simulink model "old_sea_controllers"  (R2012b)
settings: Solver=ode45  StartTime=0.0  StopTime=10.0  RelTol=1e-3
values from neighbouring files (symbols this model uses):
  sample_time = 1/update_freq    (= 0.001)    [init_umich_2d_walking.m]
undefined symbols (not defined in the file or in its folder): DiscIntNeverNeededParam, i_limit_sea_position, k_leg_spring, kd_sea_position, ki_sea_position, ki_sea_torque, kp_sea_position, kp_sea_torque, LEG_MTR_MAX_TORQUE, virtual_spring_damping
settings Model: Creator=wmartin  LastModifiedBy=wmartin

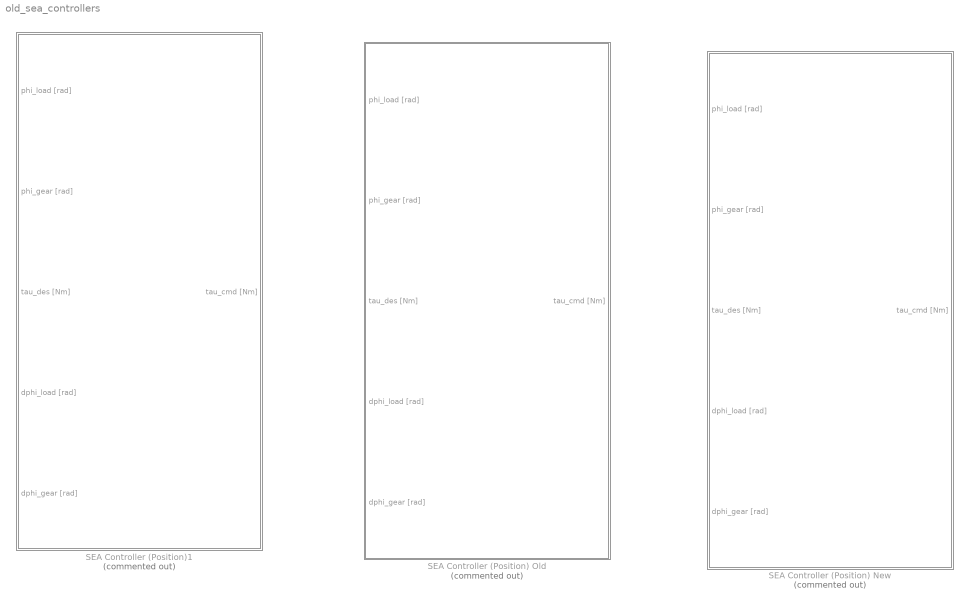
== system old_sea_controllers ==
  SEA Controller (Position) New : Subsystem  Commented=on
  SEA Controller (Position) Old : Subsystem  Commented=on
  SEA Controller (Position)1 : Subsystem  Commented=on

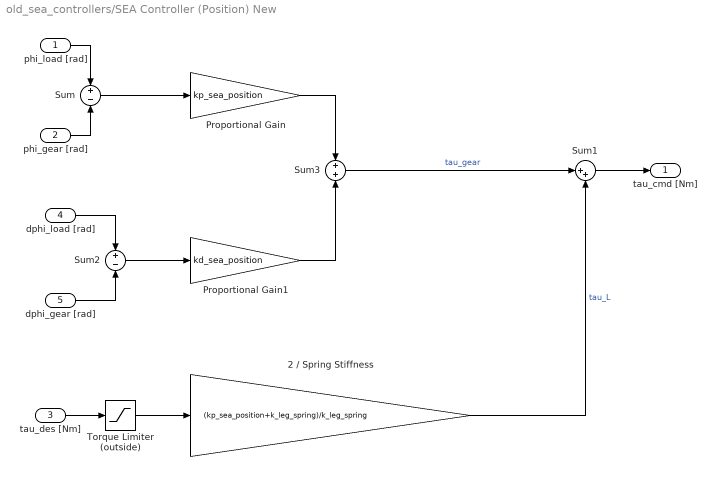
== system old_sea_controllers/SEA Controller (Position) New ==
  phi_load [rad] : Inport
  phi_gear [rad] : Inport  Port=2
  tau_des [Nm] : Inport  Port=3
  dphi_load [rad] : Inport  Port=4
  dphi_gear [rad] : Inport  Port=5
  2 / Spring Stiffness : Gain  Gain=(kp_sea_position+k_leg_spring)/k_leg_spring
  Proportional Gain : Gain  Description=xPCTag(1)=kp_sea_position;  Gain=kp_sea_position
  Proportional Gain1 : Gain  Description=xPCTag(1)=kd_sea_position;  Gain=kd_sea_position
  Sum : Sum  Inputs=+-
  Sum1 : Sum  Inputs=|++
  Sum2 : Sum  Inputs=+-
  Sum3 : Sum
  "Torque Limiter (outside) " : Saturate  UpperLimit=LEG_MTR_MAX_TORQUE  LowerLimit=-LEG_MTR_MAX_TORQUE
  tau_cmd [Nm] : Outport
  wires:
  "Torque Limiter (outside) "/1 -> 2 / Spring Stiffness/1
  tau_des [Nm]/1 -> "Torque Limiter (outside) "/1
  2 / Spring Stiffness/1 -> Sum1/2  "tau_L"
  Sum/1 -> Proportional Gain/1
  Proportional Gain/1 -> Sum3/1
  Sum3/1 -> Sum1/1  "tau_gear"
  Proportional Gain1/1 -> Sum3/2
  phi_load [rad]/1 -> Sum/1
  dphi_load [rad]/1 -> Sum2/1
  dphi_gear [rad]/1 -> Sum2/2
  Sum2/1 -> Proportional Gain1/1
  phi_gear [rad]/1 -> Sum/2
  Sum1/1 -> tau_cmd [Nm]/1

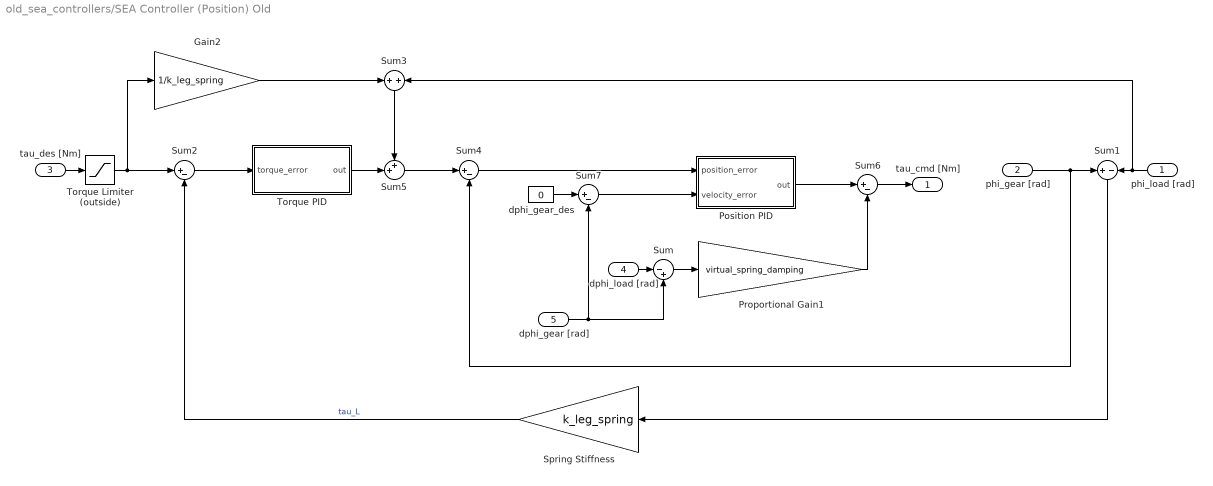
== system old_sea_controllers/SEA Controller (Position) Old ==
  phi_load [rad] : Inport
  phi_gear [rad] : Inport  Port=2
  tau_des [Nm] : Inport  Port=3
  dphi_load [rad] : Inport  Port=4
  dphi_gear [rad] : Inport  Port=5
  Gain2 : Gain  Gain=1/k_leg_spring
  Position PID : Subsystem
  Proportional Gain1 : Gain  Description=xPCTag(1)=virtual_spring_damping;  Gain=virtual_spring_damping
  Spring Stiffness : Gain  Gain=k_leg_spring
  Sum : Sum  Inputs=|-+
  Sum1 : Sum  Inputs=+-
  Sum{2,4,6..7} (4 alike) : Sum  Inputs=|+-
  Sum3 : Sum  Inputs=+|+
  Sum5 : Sum  Inputs=++|
  "Torque Limiter (outside) " : Saturate  UpperLimit=LEG_MTR_MAX_TORQUE  LowerLimit=-LEG_MTR_MAX_TORQUE
  Torque PID : Subsystem
  dphi_gear_des : Constant  Value=0
  tau_cmd [Nm] : Outport
  wires:
  dphi_gear [rad]/1 -> Sum/2, Sum7/2
  dphi_gear_des/1 -> Sum7/1
  Sum6/1 -> tau_cmd [Nm]/1
  Proportional Gain1/1 -> Sum6/2
  Sum/1 -> Proportional Gain1/1
  Sum7/1 -> Position PID/2(velocity_error)
  phi_gear [rad]/1 -> Sum1/1, Sum4/2
  Sum4/1 -> Position PID/1(position_error)
  Position PID/1(out) -> Sum6/1
  "Torque Limiter (outside) "/1 -> Sum2/1, Gain2/1
  Gain2/1 -> Sum3/1
  Spring Stiffness/1 -> Sum2/2  "tau_L"
  tau_des [Nm]/1 -> "Torque Limiter (outside) "/1
  Sum2/1 -> Torque PID/1(torque_error)
  Sum1/1 -> Spring Stiffness/1
  phi_load [rad]/1 -> Sum1/2, Sum3/2
  Sum3/1 -> Sum5/1
  Sum5/1 -> Sum4/1
  Torque PID/1(out) -> Sum5/2
  dphi_load [rad]/1 -> Sum/1

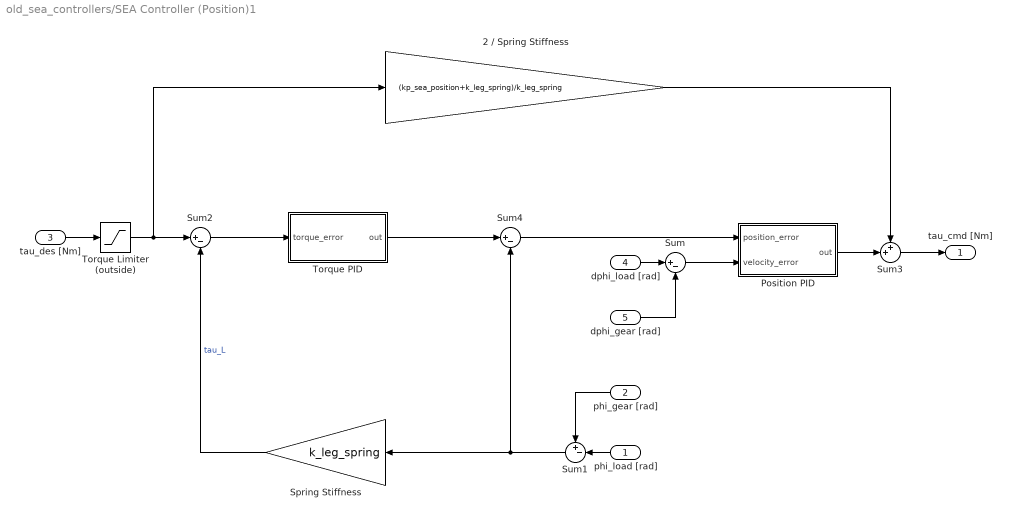
== system old_sea_controllers/SEA Controller (Position)1 ==
  phi_load [rad] : Inport
  phi_gear [rad] : Inport  Port=2
  tau_des [Nm] : Inport  Port=3
  dphi_load [rad] : Inport  Port=4
  dphi_gear [rad] : Inport  Port=5
  2 / Spring Stiffness : Gain  Gain=(kp_sea_position+k_leg_spring)/k_leg_spring
  Position PID : Subsystem
  Spring Stiffness : Gain  Gain=k_leg_spring
  Sum : Sum  Inputs=|+-
  Sum1 : Sum  Inputs=+-|
  Sum2 : Sum  Inputs=|+-
  Sum3 : Sum  Inputs=++|
  Sum4 : Sum  Inputs=|+-
  "Torque Limiter (outside) " : Saturate  UpperLimit=LEG_MTR_MAX_TORQUE  LowerLimit=-LEG_MTR_MAX_TORQUE
  Torque PID : Subsystem
  tau_cmd [Nm] : Outport
  wires:
  phi_load [rad]/1 -> Sum1/2
  phi_gear [rad]/1 -> Sum1/1
  Sum3/1 -> tau_cmd [Nm]/1
  2 / Spring Stiffness/1 -> Sum3/1
  Torque PID/1(out) -> Sum4/1
  Position PID/1(out) -> Sum3/2
  dphi_gear [rad]/1 -> Sum/2
  Sum/1 -> Position PID/2(velocity_error)
  Sum4/1 -> Position PID/1(position_error)
  "Torque Limiter (outside) "/1 -> 2 / Spring Stiffness/1, Sum2/1
  Spring Stiffness/1 -> Sum2/2  "tau_L"
  tau_des [Nm]/1 -> "Torque Limiter (outside) "/1
  Sum2/1 -> Torque PID/1(torque_error)
  Sum1/1 -> Sum4/2, Spring Stiffness/1
  dphi_load [rad]/1 -> Sum/1

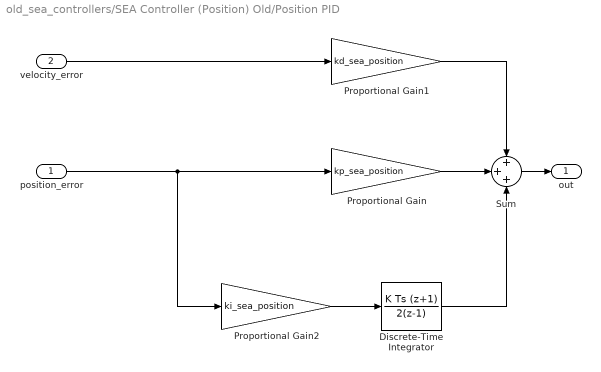
== system old_sea_controllers/SEA Controller (Position) Old/Position PID ==
  position_error : Inport
  velocity_error : Inport  Port=2
  Discrete-Time Integrator : DiscreteIntegrator  IntegratorMethod=Integration: Trapezoidal  SampleTime=sample_time  LimitOutput=on  UpperSaturationLimit=i_limit_sea_position  LowerSaturationLimit=-i_limit_sea_position  ICPrevOutput=DiscIntNeverNeededParam  ICPrevScaledInput=DiscIntNeverNeededParam
  Proportional Gain : Gain  Description=xPCTag(1)=kp_sea_position;  Gain=kp_sea_position
  Proportional Gain1 : Gain  Description=xPCTag(1)=kd_sea_position;  Gain=kd_sea_position
  Proportional Gain2 : Gain  Description=xPCTag(1)=ki_sea_position;  Gain=ki_sea_position
  Sum : Sum  Inputs=+++
  out : Outport
  wires:
  Proportional Gain1/1 -> Sum/1
  Sum/1 -> out/1
  position_error/1 -> Proportional Gain/1, Proportional Gain2/1
  Proportional Gain/1 -> Sum/2
  Proportional Gain2/1 -> Discrete-Time Integrator/1
  Discrete-Time Integrator/1 -> Sum/3
  velocity_error/1 -> Proportional Gain1/1

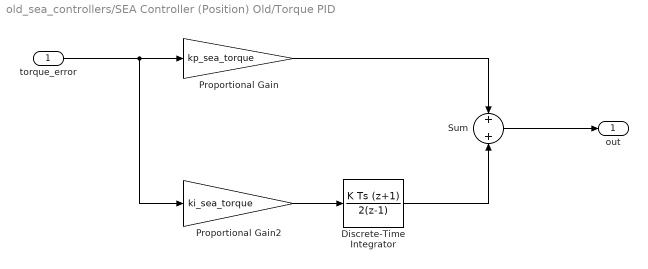
== system old_sea_controllers/SEA Controller (Position) Old/Torque PID ==
  torque_error : Inport
  Discrete-Time Integrator : DiscreteIntegrator  IntegratorMethod=Integration: Trapezoidal  SampleTime=sample_time  LimitOutput=on  UpperSaturationLimit=i_limit_sea_position  LowerSaturationLimit=-i_limit_sea_position  ICPrevOutput=DiscIntNeverNeededParam  ICPrevScaledInput=DiscIntNeverNeededParam
  Proportional Gain : Gain  Description=xPCTag(1)=kp_sea_torque;  Gain=kp_sea_torque
  Proportional Gain2 : Gain  Description=xPCTag(1)=ki_sea_torque;  Gain=ki_sea_torque
  Sum : Sum
  out : Outport
  wires:
  Discrete-Time Integrator/1 -> Sum/2
  Sum/1 -> out/1
  Proportional Gain2/1 -> Discrete-Time Integrator/1
  Proportional Gain/1 -> Sum/1
  torque_error/1 -> Proportional Gain/1, Proportional Gain2/1

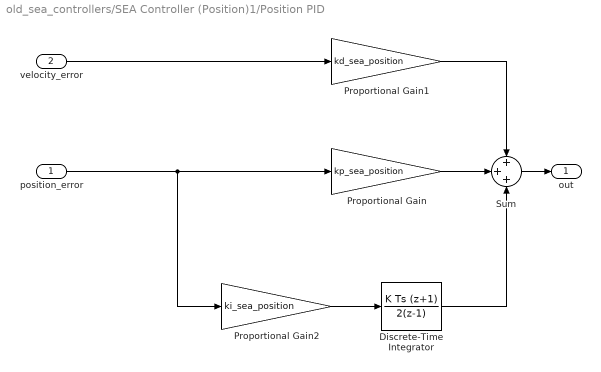
== system old_sea_controllers/SEA Controller (Position)1/Position PID ==
  position_error : Inport
  velocity_error : Inport  Port=2
  Discrete-Time Integrator : DiscreteIntegrator  IntegratorMethod=Integration: Trapezoidal  SampleTime=sample_time  LimitOutput=on  UpperSaturationLimit=i_limit_sea_position  LowerSaturationLimit=-i_limit_sea_position  ICPrevOutput=DiscIntNeverNeededParam  ICPrevScaledInput=DiscIntNeverNeededParam
  Proportional Gain : Gain  Description=xPCTag(1)=kp_sea_position;  Gain=kp_sea_position
  Proportional Gain1 : Gain  Description=xPCTag(1)=kd_sea_position;  Gain=kd_sea_position
  Proportional Gain2 : Gain  Description=xPCTag(1)=ki_sea_position;  Gain=ki_sea_position
  Sum : Sum  Inputs=+++
  out : Outport
  wires:
  Proportional Gain1/1 -> Sum/1
  Sum/1 -> out/1
  position_error/1 -> Proportional Gain/1, Proportional Gain2/1
  Proportional Gain/1 -> Sum/2
  Proportional Gain2/1 -> Discrete-Time Integrator/1
  Discrete-Time Integrator/1 -> Sum/3
  velocity_error/1 -> Proportional Gain1/1

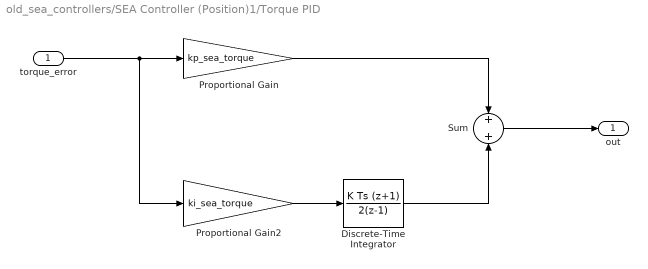
== system old_sea_controllers/SEA Controller (Position)1/Torque PID ==
  torque_error : Inport
  Discrete-Time Integrator : DiscreteIntegrator  IntegratorMethod=Integration: Trapezoidal  SampleTime=sample_time  LimitOutput=on  UpperSaturationLimit=i_limit_sea_position  LowerSaturationLimit=-i_limit_sea_position  ICPrevOutput=DiscIntNeverNeededParam  ICPrevScaledInput=DiscIntNeverNeededParam
  Proportional Gain : Gain  Description=xPCTag(1)=kp_sea_torque;  Gain=kp_sea_torque
  Proportional Gain2 : Gain  Description=xPCTag(1)=ki_sea_torque;  Gain=ki_sea_torque
  Sum : Sum
  out : Outport
  wires:
  Discrete-Time Integrator/1 -> Sum/2
  Sum/1 -> out/1
  Proportional Gain2/1 -> Discrete-Time Integrator/1
  Proportional Gain/1 -> Sum/1
  torque_error/1 -> Proportional Gain/1, Proportional Gain2/1
